simulink model "osci"  (R2023b)
settings: Solver=FixedStepAuto  StartTime=0.0  StopTime=Inf  RelTol=1e-3  EnableMultiTasking=on
libraries: canmsglib x1, raspberrypiCommlib x1
settings Model: ExtModeTrigDuration=2  Creator=aaron  LastModifiedBy=aaron
settings SolverCC: PositivePriorityOrder=on
settings OptimizationCC: EnhancedBackFolding=on  PassReuseOutputArgsAs=Individual arguments  ZeroExternalMemoryAtStartup=off  ZeroInternalMemoryAtStartup=off  MaxStackSize=64  OptimizeBlockOrder=speed  DifferentSizesBufferReuse=on  OptimizationCustomize=off  EfficientTunableParamExpr=on
settings DebuggingCC: ParameterTunabilityLossMsg=error
settings HardwareCC: ProdBitPerPointer=32  ProdBitPerSizeT=32  ProdBitPerPtrDiffT=32  ProdLargestAtomicInteger=Long  ProdLargestAtomicFloat=Double  ProdWordSize=32  ProdLongLongMode=on  ProdHWDeviceType=ARM Compatible->ARM Cortex
settings RTWCC: Description=Embedded Coder  SystemTargetFile=ert.tlc  HardwareBoard=Raspberry Pi  TLCOptions="-aInlineSetEventsForThisBaseRateFcn=TLC_FALSE -aSuppressMultiTaskScheduler=TLC_FALSE  -aRateBasedStepFcn=0"  TemplateMakefile=ert_default_tmf  Toolchain=GNU GCC Embedded Linux  BuildConfiguration=Faster Runs
settings CodeAppCC: ForceParamTrailComments=on  IgnoreCustomStorageClasses=off  OperatorAnnotations=on  SimulinkDataObjDesc=on  SFDataObjDesc=on  InsertBlockDesc=on
settings ERTTargetCC: SupportVariableSizeSignals=on  ExtModeTransport=2  ExtModeStaticAlloc=on  ExtModeMexFile=ext_xcp  ExtModeIntrfLevel=Level2 - Open

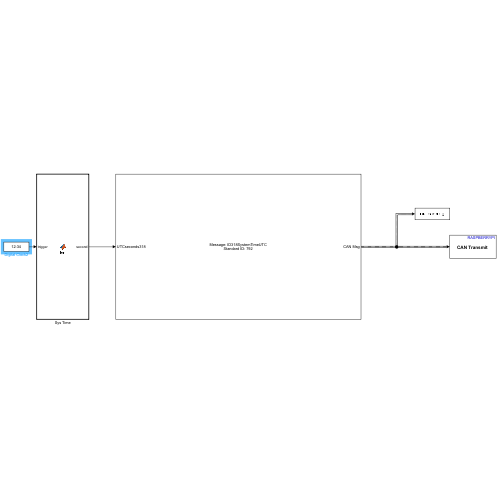
[thumbnail: Simulink's stored preview of the top-level diagram]
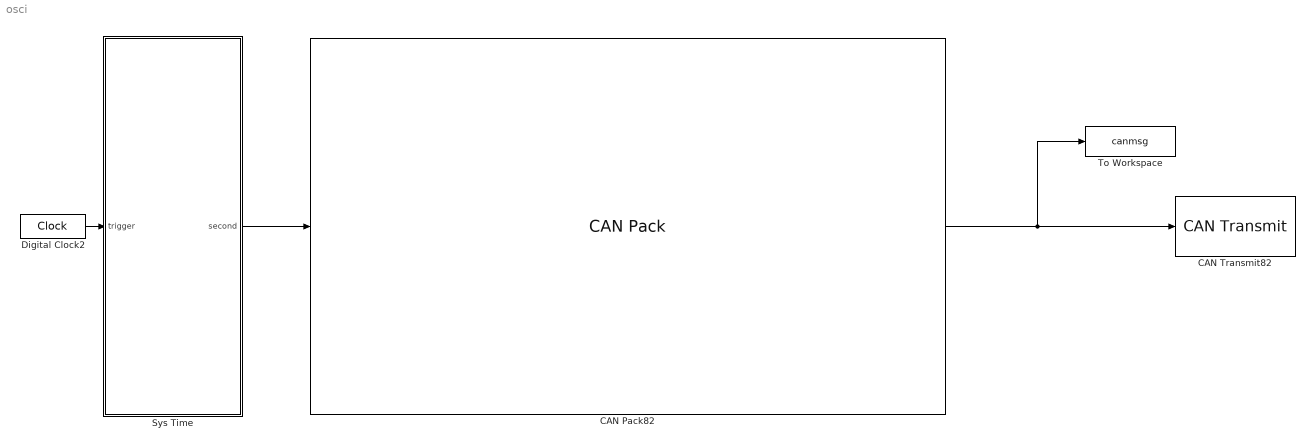
== system osci ==
  CAN Pack82 : canmsglib/CAN Pack  CANdbFile=C:\Users\aaron\OneDrive - Loughborough University\Work\Part D\FYP\tesla sniffing\Model3CAN.dbc  MsgList=ID318SystemTimeUTC  MsgName=ID318SystemTimeUTC  MsgIDType=Standard (11-bit identifier)  MsgIdentifier=792  MsgLength=1  Remote=off  ApplyMinMax=off  BusOutput=on  SignalInfo={ 'UTCseconds318', '0', '8', 'LE', 'unsigned', 'Standard', '0', '1', '0', '-Inf', 'Inf' }
      settings: LibrarySourceBlock=canlib/CAN Pack  DataFormat=manually specified signals
  CAN Transmit82 : raspberrypiCommlib/CAN Transmit  DeviceID=can0  SetupCAN=off  TypeofCAN=Real  InputDataType=CAN Msg  BlockingMode_=off  BlockTimeout_=1  OutputStatus=off  IdentifierType=Standard (11-bit identifier)  MessageId=100  MsgLength=8  RemoteFrame=off  SimulateUsing=Code generation
  Digital Clock2 : DigitalClock
  Sys Time : MATLAB Function  TreatAsAtomicUnit=on
  To Workspace : ToWorkspace  VariableName=canmsg  SaveFormat=Timeseries  SampleTime=-1
  wires:
  Digital Clock2/1 -> Sys Time/1(trigger)
  Sys Time/1(second) -> CAN Pack82/1
  CAN Pack82/1 -> To Workspace/1, CAN Transmit82/1

== matlab function osci/Sys Time ==
  data: trigger input; second output
function second  = fcn(trigger)

% function [day, hour, minute, month, second, year] = fcn(trigger)

utcTime = datetime('now');

% day = utcTime.Day;
% hour = utcTime.Hour;
% minute = utcTime.Minute;
% month = utcTime.Month;
second = utcTime.Second;
% year = utcTime.Year;
